simulink model "Sense_K"  (R2016b)
settings: Solver=FixedStepAuto  StartTime=0.0  StopTime=tF  FixedStep=0.01  RelTol=1e-3
values from neighbouring files (symbols this model uses):
  K = K_r(i)    [Proj_1a.m]    (also in Proj_1b.m; Proj_5.m = K_i(i))
  K_dth = 0.05    [Proj_1b.m]    (also in Proj_5.m = -0.04; parameters.m = 0.05*sgn)
  M_d = M_d_r(i)    [Proj_7.m]    (also in parameters.m = 200*sgn)
  T_m = 120    [parameters.m]
  tau = tau_i(i)    [Proj_4.m]    (also in parameters.m = 0.05)
settings Model: Creator=Daniel  LastModifiedBy=Daniel

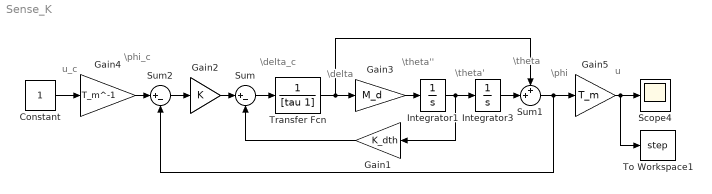
== system Sense_K ==
  note: \theta'
  note: \theta''
  note: \theta
  note: \delta
  note: \delta_c
  note: \phi_c
  note: \phi
  note: u
  note: u_c
  Constant : Constant
  Gain1 : Gain  Gain=K_dth
  Gain2 : Gain  Gain=K
  Gain3 : Gain  Gain=M_d
  Gain4 : Gain  Gain=T_m^-1
  Gain5 : Gain  Gain=T_m
  Integrator1 : Integrator
  Integrator3 : Integrator
  Scope4 : Scope
  Sum : Sum  Inputs=|+-
  Sum1 : Sum  Inputs=++|
  Sum2 : Sum  Inputs=|+-
  To Workspace1 : ToWorkspace  VariableName=step  SaveFormat=Timeseries  SampleTime=-1
  Transfer Fcn : TransferFcn  Denominator=[tau 1]
  wires:
  Gain1/1 -> Sum/2
  Sum/1 -> Transfer Fcn/1
  Gain2/1 -> Sum/1
  Transfer Fcn/1 -> Sum1/1, Gain3/1
  Sum1/1 -> Sum2/2, Gain5/1
  Gain3/1 -> Integrator1/1
  Integrator1/1 -> Integrator3/1, Gain1/1
  Integrator3/1 -> Sum1/2
  Sum2/1 -> Gain2/1
  Gain5/1 -> Scope4/1, To Workspace1/1
  Constant/1 -> Gain4/1
  Gain4/1 -> Sum2/1
